simulink model "reichardt_array_EMD_2"  (R2019a)
settings: Solver=ode45  StartTime=0.0  StopTime=setStopTime  FixedStep=0.0005  RelTol=1e-3  EnableMultiTasking=on
model workspace (MAT data in the model file):
  bodyAmp = 0
  bodyPhase = 0
  freq = 2.96243790602
  headAmp = 0
  headPhase = 0
  imageData = [0.00228480667088 0.00685422825671 0.0114230745906 0.0159909622235 0.0205575077854 0.0251223280162 0.0296850397975 0.0342452601838 0.0388026064343 0.0433566960441 0.0479071467754 0.0524535766893 ... (8204 elements, 1x8204)]
  outputTimeList = [2.12095088792 2.1421603968 2.16336990568 2.18457941456 2.20578892344 2.22699843232 2.2482079412 2.26941745007 2.29062695895 2.31183646783 2.33304597671 2.35425548559 2.37546499447 2.39667450335 2.41788401223 2.43909352111 2.46030302999 2.48151253887 2.50272204775 2.52393155663 2.5451410655 2.56635057438 2.58756008326 2.60876959214 2.62997910102 2.6511886099 2.67239811878 2.69360762766 2.71481713654 2.73602664542 2.7572361543 2.77844566318 2.79965517205 2.82086468093 2.84207418981 2.86328369869 2.88449320757 2.90570271645 2.92691222533 2.94812173421 2.96933124309 2.99054075197 3.01175026085 3.03295976973 3.05416927861 3.07537878748 3.09658829636 3.11779780524 3.13900731412 3.160216823 3.18142633188 3.20263584076 3.22384534964 3.24505485852 3.2662643674 3.28747387628 3.30868338516 3.32989289403 3.35110240291 3.37231191179 3.39352142067 3.41473092955 3.43594043843 3.45714994731 3.47835945619 3.49956896507 3.52077847395 3.54198798283 3.56319749171 3.58440700059 3.60561650946 3.62682601834 3.64803552722 3.6692450361 3.69045454498 3.71166405386 3.73287356274 3.75408307162 3.7752925805 3.79650208938 3.81771159826 3.83892110714 3.86013061601 3.88134012489 3.90254963377 3.92375914265 3.94496865153 3.96617816041 3.98738766929 4.00859717817 4.02980668705 4.05101619593 4.07222570481 4.09343521369 4.11464472257 4.13585423144 4.15706374032 4.1782732492 4.19948275808 4.22069226696 4.24190177584]
  setStopTime = 4.24190177584
  stimAmp = 15
  temporalFilt = 60
  timeConstant = 0.035
libraries: visionsources x1
(part 1 of 2)
settings Model: SimulationMode=accelerator  Creator=Shane  LastModifiedBy=BC
settings DataIOCC: SaveFormat=Array  OutputOption=SpecifiedOutputTimes  OutputTimes=outputTimeList
settings OptimizationCC: ExpressionDepthLimit=2147483647  EfficientMapNaN2IntZero=off  SimCompilerOptimization=on
settings DebuggingCC: UnderspecifiedInitializationDetection=Classic  MergeDetectMultiDrivingBlocksExec=none  FcnCallInpInsideContextMsg=warning  StateNameClashWarn=warning  SFUnexpectedBacktrackingDiag=warning  SFNoUnconditionalDefaultTransitionDiag=warning  SFExecutionAtInitializationDiag=none  ArithmeticOperatorsInVariantConditions=warning
settings HardwareCC: ProdBitPerPointer=32  ProdBitPerSizeT=32  ProdBitPerPtrDiffT=32  ProdLargestAtomicFloat=None  ProdIntDivRoundTo=Undefined  ProdEndianess=Unspecified  ProdWordSize=32  ProdHWDeviceType=32-bit Generic  TargetBitPerPointer=64  TargetBitPerSizeT=64  TargetBitPerPtrDiffT=64  TargetLongLongMode=on  TargetIntDivRoundTo=Zero  TargetEndianess=LittleEndian  TargetWordSize=64  TargetHWDeviceType=MATLAB Host  ProdEqTarget=off
settings ModelReferenceCC: PropagateSignalLabelsOutOfModel=off
settings SFSimCC: SimUseLocalCustomCode=off
settings RTWCC: SystemTargetFile=accel.tlc  TemplateMakefile=accel_default_tmf  RTWVerbose=off
settings CodeAppCC: MaxIdLength=128
settings STFCustomTargetCC: ConcurrentExecutionCompliant=on  MATLABClassNameForMDSCustomization=Simulink.SoftwareTarget.TargetSpecificTriggerConfigurationBase  SystemTargetFile=accel.tlc
settings ConfigComp: CovMetricSettings=dw  CovHtmlReporting=on  CovSaveCumulativeToWorkspaceVar=on  CovSaveSingleToWorkspaceVar=on  CovExternalEMLEnable=off

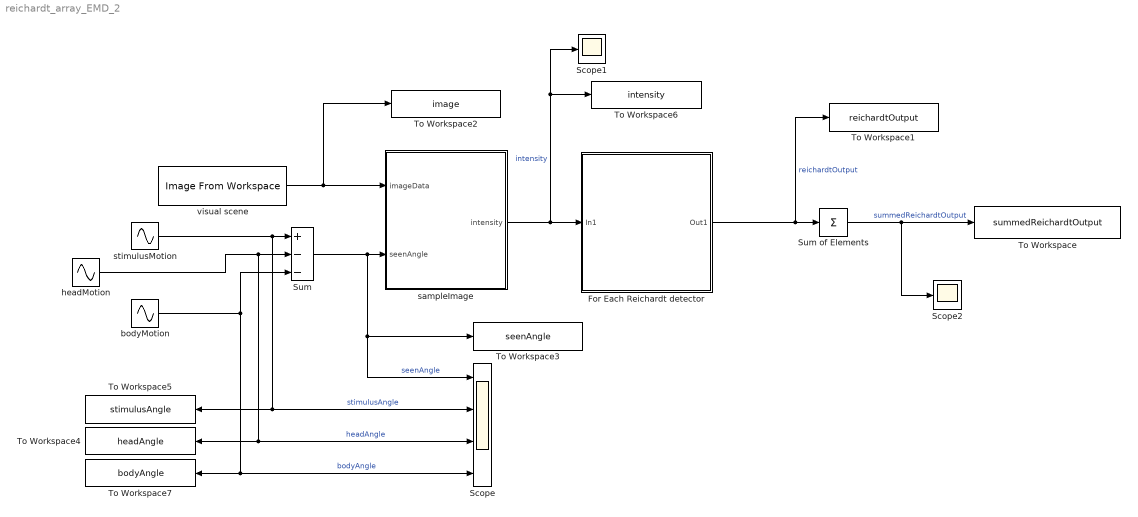
== system reichardt_array_EMD_2 ==
  For Each Reichardt detector : Subsystem  TreatAsAtomicUnit=on
  Scope : Scope  NumInputPorts=4
  Scope1 : Scope
  Scope2 : Scope
  Sum : Sum  Inputs=+--
  Sum of Elements : Sum  Inputs=+
  To Workspace : ToWorkspace  VariableName=summedReichardtOutput  SaveFormat=Timeseries  SampleTime=-1
  To Workspace1 : ToWorkspace  VariableName=reichardtOutput  SaveFormat=Timeseries  SampleTime=-1
  To Workspace2 : ToWorkspace  VariableName=image  SaveFormat=Timeseries  SampleTime=-1
  To Workspace3 : ToWorkspace  VariableName=seenAngle  SaveFormat=Timeseries  SampleTime=-1
  To Workspace4 : ToWorkspace  VariableName=headAngle  SaveFormat=Timeseries  SampleTime=-1
  To Workspace5 : ToWorkspace  VariableName=stimulusAngle  SaveFormat=Timeseries  SampleTime=-1
  To Workspace6 : ToWorkspace  VariableName=intensity  SaveFormat=Timeseries  SampleTime=-1
  To Workspace7 : ToWorkspace  VariableName=bodyAngle  SaveFormat=Timeseries  SampleTime=-1
  bodyMotion : Sin  Amplitude=bodyAmp  Frequency=freq  Phase=bodyPhase  SampleTime=0
  headMotion : Sin  Amplitude=headAmp  Frequency=freq  Phase=headPhase  SampleTime=0
  sampleImage : MATLAB Function  TreatAsAtomicUnit=on
  stimulusMotion : Sin  Amplitude=stimAmp  Frequency=freq  SampleTime=0
  visual scene : visionsources/Image From Workspace  Tag=vipblks_nd  ImageValue=imageData  Ts=inf  imagePorts=One multidimensional signal  OutPortLabels=R|G|B  ImageDataType=double  Signed=on  WordLength=16  sdImageDataType=sfix(16)  FractionLengthMode=User-defined  FractionLength=15
      settings: SourceProductName=Computer Vision Toolbox  SourceProductBaseCode=VP
  wires:
  For Each Reichardt detector/1(Out1) -> To Workspace1/1, Sum of Elements/1  "reichardtOutput"
  Sum of Elements/1 -> Scope2/1, To Workspace/1  "summedReichardtOutput"
  sampleImage/1(intensity) -> Scope1/1, To Workspace6/1, For Each Reichardt detector/1(In1)  "intensity"
  visual scene/1 -> To Workspace2/1, sampleImage/1(imageData)
  stimulusMotion/1 -> To Workspace5/1, Scope/2, Sum/1  "stimulusAngle"
  headMotion/1 -> To Workspace4/1, Scope/3, Sum/2  "headAngle"
  Sum/1 -> Scope/1, To Workspace3/1, sampleImage/2(seenAngle)  "seenAngle"
  bodyMotion/1 -> Sum/3, To Workspace7/1, Scope/4  "bodyAngle"
